simulink model "Sistema_Bioreactor"  (R2017a)
settings: Solver=VariableStepAuto  StartTime=0.0  StopTime=200  RelTol=1e-3
values from neighbouring files (symbols this model uses):
  Da1 = 1    [Bioreactor.m]
  Da2 = 1    [Bioreactor.m]
settings Model: Creator=franj  LastModifiedBy=franj

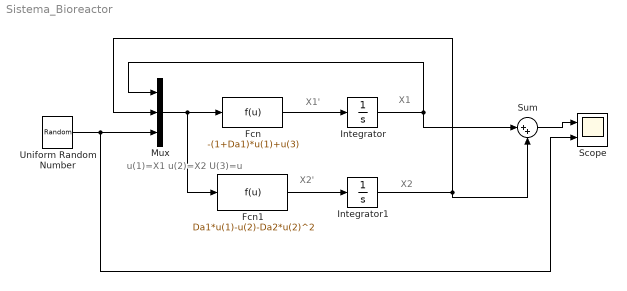
== system Sistema_Bioreactor ==
  note: u(1)=X1
      | u(2)=X2
      | U(3)=u
  note: X2
  note: X2'
  note: X1
  note: X1'
  Fcn : Fcn  Expr=-(1+Da1)*u(1)+u(3)
  Fcn1 : Fcn  Expr=Da1*u(1)-u(2)-Da2*u(2)^2
  Integrator : Integrator
  Integrator1 : Integrator
  Mux : Mux  Inputs=3
  Scope : Scope  NumInputPorts=2
  Sum : Sum  Inputs=|++
  Uniform Random Number : UniformRandomNumber  Minimum=0  Maximum=5  SampleTime=10
  wires:
  Fcn1/1 -> Integrator1/1
  Fcn/1 -> Integrator/1
  Mux/1 -> Fcn1/1, Fcn/1
  Integrator1/1 -> Sum/2, Mux/2
  Integrator/1 -> Mux/1, Sum/1
  Uniform Random Number/1 -> Scope/2, Mux/3
  Sum/1 -> Scope/1
